simulink model "Utkarsh_2005574_R_W1_P9"  (R2021a)
settings: Solver=VariableStepAuto  StartTime=0.0  StopTime=0.5  RelTol=1e-3
undefined symbols (not defined in the file): Dm, J, Lam, Lss, P, rs, Tm, Ts, Vdc
settings Model: Creator=Utkarsh Anand  LastModifiedBy=Utkarsh Anand

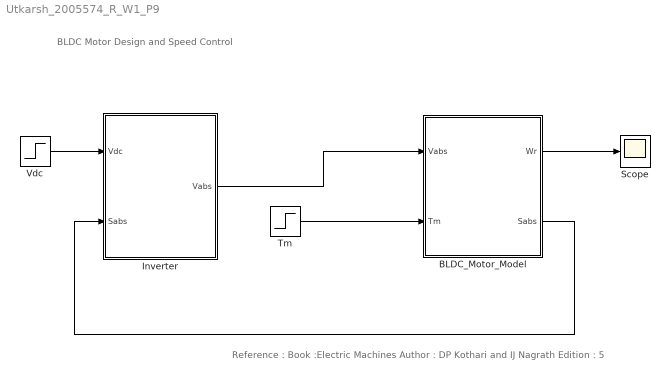
== system Utkarsh_2005574_R_W1_P9 ==
  note: Reference :
      | Book :Electric Machines
      | Author : DP Kothari and IJ Nagrath
      | Edition : 5
  note: BLDC Motor Design and Speed Control
  BLDC_Motor_Model : Subsystem
  Inverter : Subsystem  TreatAsAtomicUnit=on
  Scope : Scope
  Tm : Step  Time=0.5  After=Tm  SampleTime=0
  Vdc : Step  Time=0.05  After=Vdc  SampleTime=0
  wires:
  BLDC_Motor_Model/2(Sabs) -> Inverter/2(Sabs)
  Tm/1 -> BLDC_Motor_Model/2(Tm)
  BLDC_Motor_Model/1(Wr) -> Scope/1
  Vdc/1 -> Inverter/1(Vdc)
  Inverter/1(Vabs) -> BLDC_Motor_Model/1(Vabs)

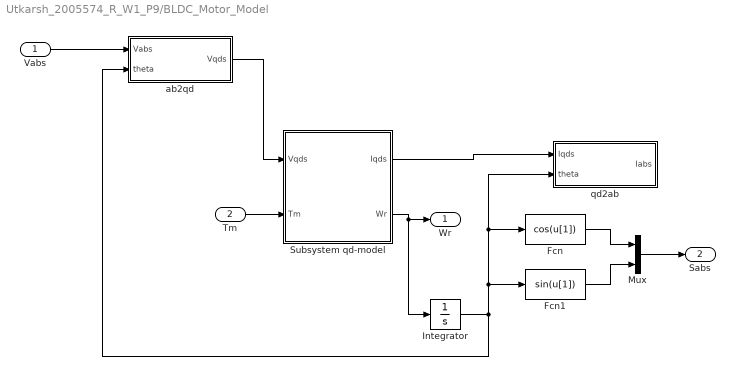
== system Utkarsh_2005574_R_W1_P9/BLDC_Motor_Model ==
  Vabs : Inport
  Tm : Inport  Port=2
  Fcn : Fcn  Expr=cos(u[1])
  Fcn1 : Fcn
  Integrator : Integrator
  Mux : Mux  Inputs=2
  Subsystem qd-model : Subsystem
  ab2qd : Subsystem
  qd2ab : Subsystem
  Wr : Outport
  Sabs : Outport  Port=2
  wires:
  Vabs/1 -> ab2qd/1(Vabs)
  ab2qd/1(" Vqds") -> Subsystem qd-model/1(Vqds)
  Tm/1 -> Subsystem qd-model/2(Tm)
  Subsystem qd-model/1(Iqds) -> qd2ab/1(Iqds)
  Subsystem qd-model/2(Wr) -> Integrator/1, Wr/1
  Integrator/1 -> ab2qd/2(theta), Fcn1/1, qd2ab/2(theta), Fcn/1
  Mux/1 -> Sabs/1
  Fcn/1 -> Mux/1
  Fcn1/1 -> Mux/2

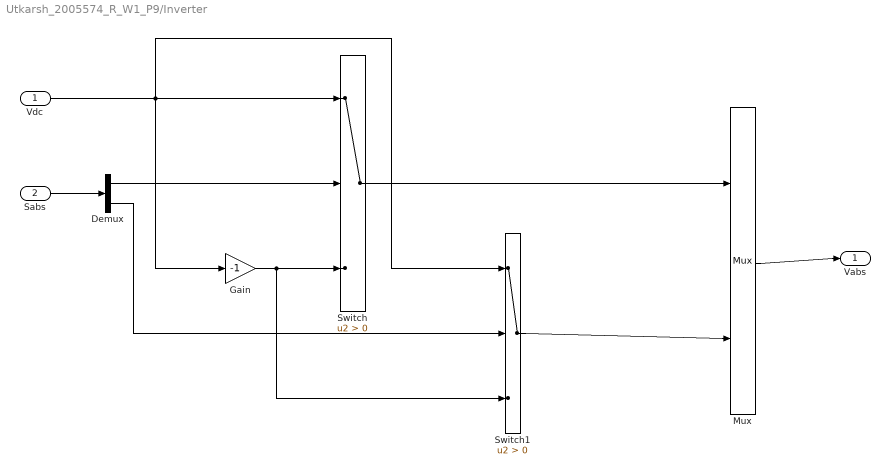
== system Utkarsh_2005574_R_W1_P9/Inverter ==
  Vdc : Inport
  Sabs : Inport  Port=2
  Demux : Demux  Outputs=2
  Gain : Gain  Gain=-1
  Mux : Mux  Inputs=2
  Switch : Switch  Criteria=u2 > Threshold
  Switch1 : Switch  Criteria=u2 > Threshold
  Vabs : Outport
  wires:
  Sabs/1 -> Demux/1
  Mux/1 -> Vabs/1
  Demux/1 -> Switch/2
  Vdc/1 -> Switch1/1, Gain/1, Switch/1
  Switch/1 -> Mux/1
  Switch1/1 -> Mux/2
  Demux/2 -> Switch1/2
  Gain/1 -> Switch/3, Switch1/3

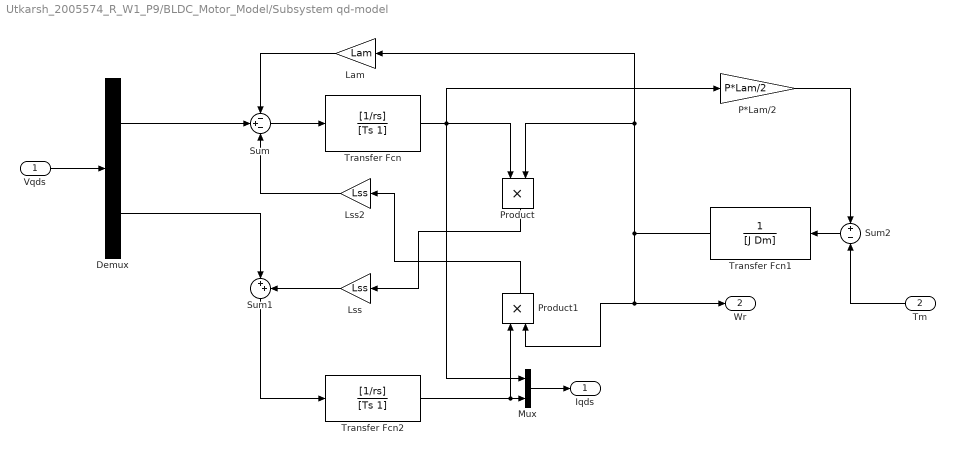
== system Utkarsh_2005574_R_W1_P9/BLDC_Motor_Model/Subsystem qd-model ==
  Vqds : Inport
  Tm : Inport  Port=2
  Demux : Demux  Outputs=2
  Lam : Gain  Gain=Lam
  Lss : Gain  Gain=Lss
  Lss2 : Gain  Gain=Lss
  Mux : Mux  Inputs=2
  P*Lam/2 : Gain  Gain=P*Lam/2
  Product : Product
  Product1 : Product
  Sum : Sum  Inputs=-+-
  Sum1 : Sum  Inputs=|++
  Sum2 : Sum  Inputs=+-
  Transfer Fcn : TransferFcn  Numerator=[1/rs]  Denominator=[Ts 1]
  Transfer Fcn1 : TransferFcn  Denominator=[J Dm]
  Transfer Fcn2 : TransferFcn  Numerator=[1/rs]  Denominator=[Ts 1]
  Iqds : Outport
  Wr : Outport  Port=2
  wires:
  Vqds/1 -> Demux/1
  Demux/1 -> Sum/2
  Demux/2 -> Sum1/1
  P*Lam/2/1 -> Sum2/1
  Tm/1 -> Sum2/2
  Lam/1 -> Sum/1
  Lss/1 -> Sum1/2
  Sum1/1 -> Transfer Fcn2/1
  Sum2/1 -> Transfer Fcn1/1
  Transfer Fcn2/1 -> Product1/1, Mux/2
  Product1/1 -> Lss2/1
  Product/1 -> Lss/1
  Transfer Fcn/1 -> Mux/1, Product/1, P*Lam/2/1
  Transfer Fcn1/1 -> Product/2, Lam/1, Product1/2, Wr/1
  Mux/1 -> Iqds/1
  Sum/1 -> Transfer Fcn/1
  Lss2/1 -> Sum/3

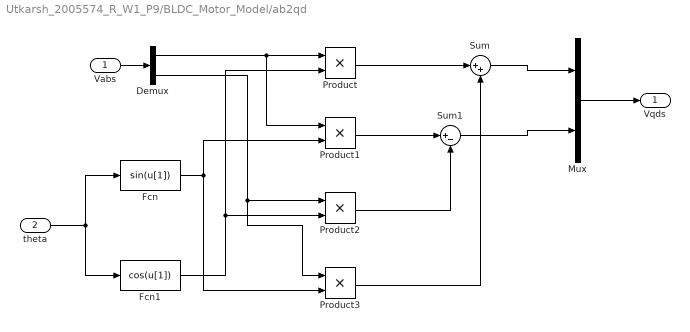
== system Utkarsh_2005574_R_W1_P9/BLDC_Motor_Model/ab2qd ==
  Vabs : Inport
  theta : Inport  Port=2
  Demux : Demux  Outputs=2
  Fcn : Fcn
  Fcn1 : Fcn  Expr=cos(u[1])
  Mux : Mux  Inputs=2
  Product{,1..3} (4 alike) : Product
  Sum : Sum  Inputs=|++
  Sum1 : Sum  Inputs=|+-
  " Vqds" : Outport
  wires:
  Vabs/1 -> Demux/1
  Mux/1 -> " Vqds"/1
  theta/1 -> Fcn/1, Fcn1/1
  Demux/1 -> Product1/1, Product/1
  Fcn1/1 -> Product2/2, Product/2
  Fcn/1 -> Product1/2, Product3/2
  Demux/2 -> Product3/1, Product2/1
  Product/1 -> Sum/1
  Product3/1 -> Sum/2
  Sum/1 -> Mux/1
  Product1/1 -> Sum1/1
  Product2/1 -> Sum1/2
  Sum1/1 -> Mux/2

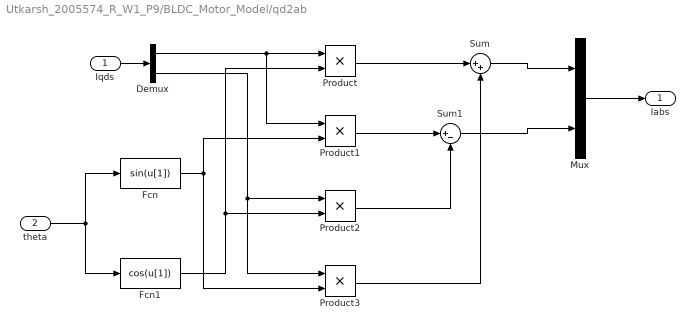
== system Utkarsh_2005574_R_W1_P9/BLDC_Motor_Model/qd2ab ==
  Iqds : Inport
  theta : Inport  Port=2
  Demux : Demux  Outputs=2
  Fcn : Fcn
  Fcn1 : Fcn  Expr=cos(u[1])
  Mux : Mux  Inputs=2
  Product{,1..3} (4 alike) : Product
  Sum : Sum  Inputs=|++
  Sum1 : Sum  Inputs=|+-
  " Iabs" : Outport
  wires:
  Iqds/1 -> Demux/1
  Mux/1 -> " Iabs"/1
  theta/1 -> Fcn/1, Fcn1/1
  Demux/1 -> Product1/1, Product/1
  Fcn1/1 -> Product2/2, Product/2
  Fcn/1 -> Product1/2, Product3/2
  Demux/2 -> Product3/1, Product2/1
  Product/1 -> Sum/1
  Product3/1 -> Sum/2
  Sum/1 -> Mux/1
  Product1/1 -> Sum1/1
  Product2/1 -> Sum1/2
  Sum1/1 -> Mux/2
